simulink model "Ball_and_Plate_Model"  (R2020a)
settings: Solver=VariableStepAuto  StartTime=0.0  StopTime=10.0  RelTol=1e-3
values from neighbouring files (symbols this model uses):
  d = 0.03    [ball_and_plate_TF.m]
  g = -9.8    [ball_and_plate_TF.m]
  J = 9.99e-6    (= 9.99e-06)    [ball_and_plate_TF.m]
  L = 1.0    (= 1)    [ball_and_plate_TF.m]
  m = 0.111    [ball_and_plate_TF.m]
  R = 0.015    [ball_and_plate_TF.m]
libraries: simulink x1
settings Model: Creator=Allan  LastModifiedBy=Allan

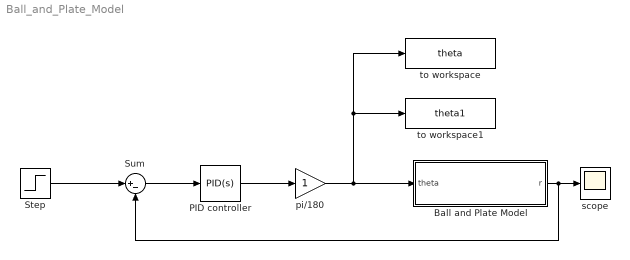
== system Ball_and_Plate_Model ==
  Ball and Plate Model : Subsystem
  PID controller : simulink/Continuous/PID Controller  Controller=PID  Form=Parallel  TimeDomain=Continuous-time  UseExternalTs=off  SampleTime=-1  IntegratorMethod=Forward Euler  FilterMethod=Forward Euler  ControllerParametersSource=internal  P=15  I=0  D=50  UseFilter=on  N=100  TunerSelectOption=Transfer Function Based (PID Tuner App)  InitialConditionSource=internal  InitialConditionForIntegrator=0  InitialConditionForFilter=0  DifferentiatorICPrevScaledInput=0  ExternalReset=none  TrackingMode=off  Kt=1  LimitOutput=off  UpperSaturationLimit=inf  LowerSaturationLimit=-inf  LinearizeAsGain=on  AntiWindupMode=none  Kb=1  POutMin=[]  POutMax=[]  IOutMin=[]  IOutMax=[]  DOutMin=[]  DOutMax=[]  NOutMin=[]  NOutMax=[]  SumOutMin=[]  SumOutMax=[]  SaturationOutMin=[]  SaturationOutMax=[]  PParamMin=[]  PParamMax=[]  IParamMin=[]  IParamMax=[]  DParamMin=[]  DParamMax=[]  NParamMin=[]  NParamMax=[]  KbParamMin=[]  KbParamMax=[]  KtParamMin=[]  KtParamMax=[]  KbOutMin=[]  KbOutMax=[]  KtOutMin=[]  KtOutMax=[]  IntegratorOutMin=[]  IntegratorOutMax=[]  FilterOutMin=[]  FilterOutMax=[]  SumI1OutMin=[]  SumI1OutMax=[]  SumI2OutMin=[]  SumI2OutMax=[]  SumI3OutMin=[]  SumI3OutMax=[]  SumI4OutMin=[]  SumI4OutMax=[]  SumDOutMin=[]  SumDOutMax=[]  DifferentiatorOutMin=[]  DifferentiatorOutMax=[]  FilterDiffOutCoefMin=[]  FilterDiffOutCoefMax=[]  ReciprocalOutMin=[]  ReciprocalOutMax=[]  SumDenOutMin=[]  SumDenOutMax=[]  SumNumOutMin=[]  SumNumOutMax=[]  DivideOutMin=[]  DivideOutMax=[]  UdiffTsProdOutMin=[]  UdiffTsProdOutMax=[]  NTsProdOutMin=[]  NTsProdOutMax=[]  UintegralTsProdOutMin=[]  UintegralTsProdOutMax=[]  UngainTsProdOutMin=[]  UngainTsProdOutMax=[]  IntegratorContinuousStateAttributes=''  IntegratorStateMustResolveToSignalObject=off  IntegratorRTWStateStorageClass=Auto  FilterContinuousStateAttributes=''  FilterStateMustResolveToSignalObject=off  FilterRTWStateStorageClass=Auto  ParallelPVariant=InternalParameters  IdealPVariant=Disabled  IVariant=InternalParameters  DVariant=InternalParameters  IntegratorVariant=Continuous  SatVariant=Disabled  AWVariant=Passthrough  PCopyVariant=Disabled  TRVariant=Disabled  FdbkBlocksVariant=Forward  IdealPFdbkVariant=Disabled  SatFdbkVariant=Disabled  DerivativeFilterVariant=ContFilter  NVariant=InternalParameters  NCopyVariant=Disabled  FilterICVariant=InternalICsFilter  IntegratorICVariant=InternalICs  ExternalResetVariant=Disabled  TRSumVariant=Passthrough  SumFdbkVariant=Disabled  SumVariant=Sum_PID  TsampFilterVariant=InternalTs  TsampNgainVariant=Passthrough  TsampIntegralVariant=Passthrough
  Step : Step  SampleTime=0
  Sum : Sum  Inputs=|+-
  pi/180 : Gain
  scope : Scope
  to workspace : ToWorkspace  VariableName=theta  SampleTime=1
  to workspace1 : ToWorkspace  VariableName=theta1  SaveFormat=Timeseries  SampleTime=-1
  wires:
  Ball and Plate Model/1(r) -> Sum/2, scope/1
  Sum/1 -> PID controller/1
  PID controller/1 -> pi/180/1
  pi/180/1 -> to workspace1/1, to workspace/1, Ball and Plate Model/1(theta)
  Step/1 -> Sum/1

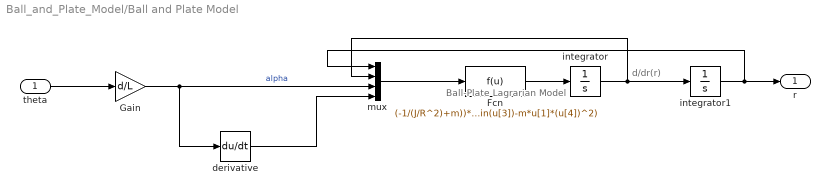
== system Ball_and_Plate_Model/Ball and Plate Model ==
  note: Ball-Plate Lagrarian Model
  note: d/dr(r)
  theta : Inport
  Fcn : Fcn  Expr=(-1/(J/R^2)+m))*(m*g*sin(u[3])-m*u[1]*(u[4])^2)
  Gain : Gain  Gain=d/L
  derivative : Derivative
  integrator : Integrator
  integrator1 : Integrator
  mux : Mux
  r : Outport
  wires:
  theta/1 -> Gain/1
  derivative/1 -> mux/4
  integrator1/1 -> mux/1, r/1
  Fcn/1 -> integrator/1
  Gain/1 -> derivative/1, mux/3  "alpha"
  integrator/1 -> mux/2, integrator1/1
  mux/1 -> Fcn/1
